simulink model "IRB140"  (R2016b)
settings: Solver=ode113  StartTime=0.0  StopTime=40  RelTol=1e-3
(part 7 of 9)

== matlab function IRB140/outer loop ==
  data: e_theta input; e_thetad input; thetadd_desired input; aq output
function aq = fcn(e_theta, e_thetad, thetadd_desired)
wn = 1;
Kp = diag(ones(6,1)*wn^2);
Kd = diag(ones(6,1)*2*wn);
aq = thetadd_desired - Kd*e_thetad - Kp*e_theta;

== matlab function IRB140/Inner loop1 ==
  data: aq input; u output
function u = fcn(aq)

D = eye(6);
V = ones(6,1);
G = ones(6,1);

u = D*aq + V + G;
